simulink model "p_controller"  (R2025b)
settings: Solver=ode45  StartTime=0.0  StopTime=2  RelTol=1e-3

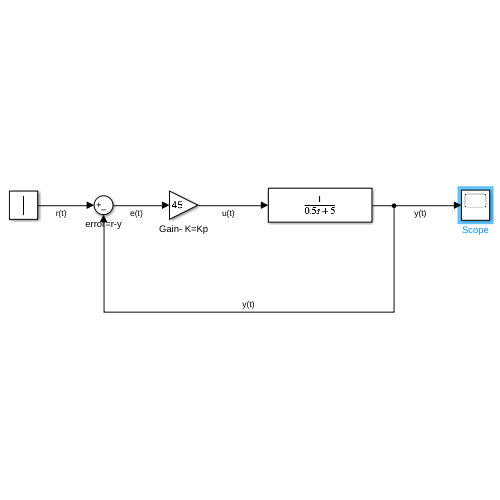
[thumbnail: Simulink's stored preview of the top-level diagram]
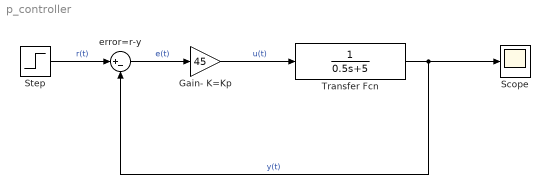
== system p_controller ==
  Gain- K=Kp : Gain  Gain=45
  Scope : Scope
      settings: ActiveDisplayYMinimum=0.614427999944724  ActiveDisplayYMaximum=1.0353620767432727
  Step : Step  Time=0  SampleTime=0
  Transfer Fcn : TransferFcn  Denominator=[0.5 5]
  error=r-y : Sum  Inputs=|+-
  wires:
  Step/1 -> error=r-y/1  "r(t)"
  error=r-y/1 -> Gain- K=Kp/1  "e(t)"
  Gain- K=Kp/1 -> Transfer Fcn/1  "u(t)"
  Transfer Fcn/1 -> error=r-y/2, Scope/1  "y(t)"
